simulink model "GMPP2"  (Simulink 8.7)
settings: Solver=ode15s  StartTime=0.0  StopTime=0.3  RelTol=1e-3
libraries: powerlib x29, simulink x13, neural x6
(part 2 of 2)

== system GMPP2/PV5/Subsystem4/Subsystem3 ==
  T : Inport
  Divide : Product  Inputs=**/
  K : Constant  Value=1.38e-23
  q : Constant  Value=1.6e-19
  Vt : Outport
  wires:
  K/1 -> Divide/1
  T/1 -> Divide/2
  q/1 -> Divide/3
  Divide/1 -> Vt/1

== system GMPP2/PV7/Subsystem/Subsystem2 ==
  T : Inport
  Subtrac : Sum  Inputs=+-
  Tn : Constant  Value=298.15
  dT : Outport
  wires:
  T/1 -> Subtrac/1
  Tn/1 -> Subtrac/2
  Subtrac/1 -> dT/1

== system GMPP2/PV7/Subsystem4/Subsystem2 ==
  T : Inport
  Subtrac : Sum  Inputs=+-
  Tn : Constant  Value=298.15
  dT : Outport
  wires:
  T/1 -> Subtrac/1
  Tn/1 -> Subtrac/2
  Subtrac/1 -> dT/1

== system GMPP2/PV7/Subsystem4/Subsystem3 ==
  T : Inport
  Divide : Product  Inputs=**/
  K : Constant  Value=1.38e-23
  q : Constant  Value=1.6e-19
  Vt : Outport
  wires:
  K/1 -> Divide/1
  T/1 -> Divide/2
  q/1 -> Divide/3
  Divide/1 -> Vt/1

== matlab function MATLAB Function ==
  data: Vg output double; V input double; P input double; GMPP output double; P_old input double; C input double; Vg_old input double; G_old input double
function [Vg,GMPP] = fcn(V,P,P_old,C,Vg_old,G_old)

%detect change on irradiance 
if C ==1 
    G_old=0 ;
    Vg_old =0;
end
if P>P_old && G_old==0    % G_old==0 => first Pmax detecting 
    GMPP=P;
    Vg = V;
elseif P>P_old && G_old~=0  % G_old~=0 => second or third Pmax detecting 
    if P> G_old
        GMPP=P;
        Vg = V;
    else
        % restore last value of Pgmmp and Vgmmp 
        GMPP=G_old;
        Vg = Vg_old;
    end
else
    GMPP=G_old;
    Vg = Vg_old;
end
